simulink model "gm_hybrid_lht_vnl"  (R2019b)
settings: Solver=FixedStepDiscrete  StartTime=0.0  StopTime=inf  FixedStep=1/120e6  RelTol=1e-3
undefined symbols (not defined in the file or in its folder): bt, height, nTheta, width
libraries: hdlsllib x252, simulink x168, hdlmdlgenlib x11, dspsrcs4 x1
(part 11 of 12)

== system gm_hybrid_lht_vnl/Hybrid LHT/Hybrid LHT Kernel/Gradient Kernel System/Hough Kernel/Look Ahead Hough/Look Ahead Hough Symmetric/Register Bank_instance2 ==
  Data In : Inport  OutDataTypeStr=int8  PortDimensions=1  SampleTime=8.33333333333333e-09
  Write Enable : Inport  Port=2  OutDataTypeStr=boolean  PortDimensions=1  SampleTime=8.33333333333333e-09
  Delay_Switch : Switch  Criteria=u2 ~= 0  Threshold=double(0)  OutDataTypeStr=int8  SampleTime=8.33333333333333e-09
  Unit Delay Enabled Synchronous_lowered : Delay  DelayLength=double(1)  InitialCondition=0  SampleTime=8.33333333333333e-09
  Data Out : Outport
  wires:
  Unit Delay Enabled Synchronous_lowered/1 -> Data Out/1, Delay_Switch/3
  Data In/1 -> Delay_Switch/1
  Write Enable/1 -> Delay_Switch/2
  Delay_Switch/1 -> Unit Delay Enabled Synchronous_lowered/1

== system gm_hybrid_lht_vnl/Hybrid LHT/Hybrid LHT Kernel/Gradient Kernel System/Hough Kernel/Look Ahead Hough/Look Ahead Hough Symmetric/Register Bank_instance20 ==
  Data In : Inport  OutDataTypeStr=int8  PortDimensions=1  SampleTime=8.33333333333333e-09
  Write Enable : Inport  Port=2  OutDataTypeStr=boolean  PortDimensions=1  SampleTime=8.33333333333333e-09
  Delay_Switch : Switch  Criteria=u2 ~= 0  Threshold=double(0)  OutDataTypeStr=int8  SampleTime=8.33333333333333e-09
  Unit Delay Enabled Synchronous_lowered : Delay  DelayLength=double(1)  InitialCondition=0  SampleTime=8.33333333333333e-09
  Data Out : Outport
  wires:
  Unit Delay Enabled Synchronous_lowered/1 -> Data Out/1, Delay_Switch/3
  Data In/1 -> Delay_Switch/1
  Write Enable/1 -> Delay_Switch/2
  Delay_Switch/1 -> Unit Delay Enabled Synchronous_lowered/1

== system gm_hybrid_lht_vnl/Hybrid LHT/Hybrid LHT Kernel/Gradient Kernel System/Hough Kernel/Look Ahead Hough/Look Ahead Hough Symmetric/Register Bank_instance21 ==
  Data In : Inport  OutDataTypeStr=int8  PortDimensions=1  SampleTime=8.33333333333333e-09
  Write Enable : Inport  Port=2  OutDataTypeStr=boolean  PortDimensions=1  SampleTime=8.33333333333333e-09
  Delay_Switch : Switch  Criteria=u2 ~= 0  Threshold=double(0)  OutDataTypeStr=int8  SampleTime=8.33333333333333e-09
  Unit Delay Enabled Synchronous_lowered : Delay  DelayLength=double(1)  InitialCondition=0  SampleTime=8.33333333333333e-09
  Data Out : Outport
  wires:
  Unit Delay Enabled Synchronous_lowered/1 -> Data Out/1, Delay_Switch/3
  Data In/1 -> Delay_Switch/1
  Write Enable/1 -> Delay_Switch/2
  Delay_Switch/1 -> Unit Delay Enabled Synchronous_lowered/1

== system gm_hybrid_lht_vnl/Hybrid LHT/Hybrid LHT Kernel/Gradient Kernel System/Hough Kernel/Look Ahead Hough/Look Ahead Hough Symmetric/Register Bank_instance22 ==
  Data In : Inport  OutDataTypeStr=int8  PortDimensions=1  SampleTime=8.33333333333333e-09
  Write Enable : Inport  Port=2  OutDataTypeStr=boolean  PortDimensions=1  SampleTime=8.33333333333333e-09
  Delay_Switch : Switch  Criteria=u2 ~= 0  Threshold=double(0)  OutDataTypeStr=int8  SampleTime=8.33333333333333e-09
  Unit Delay Enabled Synchronous_lowered : Delay  DelayLength=double(1)  InitialCondition=0  SampleTime=8.33333333333333e-09
  Data Out : Outport
  wires:
  Unit Delay Enabled Synchronous_lowered/1 -> Data Out/1, Delay_Switch/3
  Data In/1 -> Delay_Switch/1
  Write Enable/1 -> Delay_Switch/2
  Delay_Switch/1 -> Unit Delay Enabled Synchronous_lowered/1

== system gm_hybrid_lht_vnl/Hybrid LHT/Hybrid LHT Kernel/Gradient Kernel System/Hough Kernel/Look Ahead Hough/Look Ahead Hough Symmetric/Register Bank_instance23 ==
  Data In : Inport  OutDataTypeStr=int8  PortDimensions=1  SampleTime=8.33333333333333e-09
  Write Enable : Inport  Port=2  OutDataTypeStr=boolean  PortDimensions=1  SampleTime=8.33333333333333e-09
  Delay_Switch : Switch  Criteria=u2 ~= 0  Threshold=double(0)  OutDataTypeStr=int8  SampleTime=8.33333333333333e-09
  Unit Delay Enabled Synchronous_lowered : Delay  DelayLength=double(1)  InitialCondition=0  SampleTime=8.33333333333333e-09
  Data Out : Outport
  wires:
  Unit Delay Enabled Synchronous_lowered/1 -> Data Out/1, Delay_Switch/3
  Data In/1 -> Delay_Switch/1
  Write Enable/1 -> Delay_Switch/2
  Delay_Switch/1 -> Unit Delay Enabled Synchronous_lowered/1

== system gm_hybrid_lht_vnl/Hybrid LHT/Hybrid LHT Kernel/Gradient Kernel System/Hough Kernel/Look Ahead Hough/Look Ahead Hough Symmetric/Register Bank_instance24 ==
  Data In : Inport  OutDataTypeStr=int8  PortDimensions=1  SampleTime=8.33333333333333e-09
  Write Enable : Inport  Port=2  OutDataTypeStr=boolean  PortDimensions=1  SampleTime=8.33333333333333e-09
  Delay_Switch : Switch  Criteria=u2 ~= 0  Threshold=double(0)  OutDataTypeStr=int8  SampleTime=8.33333333333333e-09
  Unit Delay Enabled Synchronous_lowered : Delay  DelayLength=double(1)  InitialCondition=0  SampleTime=8.33333333333333e-09
  Data Out : Outport
  wires:
  Unit Delay Enabled Synchronous_lowered/1 -> Data Out/1, Delay_Switch/3
  Data In/1 -> Delay_Switch/1
  Write Enable/1 -> Delay_Switch/2
  Delay_Switch/1 -> Unit Delay Enabled Synchronous_lowered/1

== system gm_hybrid_lht_vnl/Hybrid LHT/Hybrid LHT Kernel/Gradient Kernel System/Hough Kernel/Look Ahead Hough/Look Ahead Hough Symmetric/Register Bank_instance25 ==
  Data In : Inport  OutDataTypeStr=int8  PortDimensions=1  SampleTime=8.33333333333333e-09
  Write Enable : Inport  Port=2  OutDataTypeStr=boolean  PortDimensions=1  SampleTime=8.33333333333333e-09
  Delay_Switch : Switch  Criteria=u2 ~= 0  Threshold=double(0)  OutDataTypeStr=int8  SampleTime=8.33333333333333e-09
  Unit Delay Enabled Synchronous_lowered : Delay  DelayLength=double(1)  InitialCondition=0  SampleTime=8.33333333333333e-09
  Data Out : Outport
  wires:
  Unit Delay Enabled Synchronous_lowered/1 -> Data Out/1, Delay_Switch/3
  Data In/1 -> Delay_Switch/1
  Write Enable/1 -> Delay_Switch/2
  Delay_Switch/1 -> Unit Delay Enabled Synchronous_lowered/1

== system gm_hybrid_lht_vnl/Hybrid LHT/Hybrid LHT Kernel/Gradient Kernel System/Hough Kernel/Look Ahead Hough/Look Ahead Hough Symmetric/Register Bank_instance26 ==
  Data In : Inport  OutDataTypeStr=int8  PortDimensions=1  SampleTime=8.33333333333333e-09
  Write Enable : Inport  Port=2  OutDataTypeStr=boolean  PortDimensions=1  SampleTime=8.33333333333333e-09
  Delay_Switch : Switch  Criteria=u2 ~= 0  Threshold=double(0)  OutDataTypeStr=int8  SampleTime=8.33333333333333e-09
  Unit Delay Enabled Synchronous_lowered : Delay  DelayLength=double(1)  InitialCondition=0  SampleTime=8.33333333333333e-09
  Data Out : Outport
  wires:
  Unit Delay Enabled Synchronous_lowered/1 -> Data Out/1, Delay_Switch/3
  Data In/1 -> Delay_Switch/1
  Write Enable/1 -> Delay_Switch/2
  Delay_Switch/1 -> Unit Delay Enabled Synchronous_lowered/1

== system gm_hybrid_lht_vnl/Hybrid LHT/Hybrid LHT Kernel/Gradient Kernel System/Hough Kernel/Look Ahead Hough/Look Ahead Hough Symmetric/Register Bank_instance27 ==
  Data In : Inport  OutDataTypeStr=int8  PortDimensions=1  SampleTime=8.33333333333333e-09
  Write Enable : Inport  Port=2  OutDataTypeStr=boolean  PortDimensions=1  SampleTime=8.33333333333333e-09
  Delay_Switch : Switch  Criteria=u2 ~= 0  Threshold=double(0)  OutDataTypeStr=int8  SampleTime=8.33333333333333e-09
  Unit Delay Enabled Synchronous_lowered : Delay  DelayLength=double(1)  InitialCondition=0  SampleTime=8.33333333333333e-09
  Data Out : Outport
  wires:
  Unit Delay Enabled Synchronous_lowered/1 -> Data Out/1, Delay_Switch/3
  Data In/1 -> Delay_Switch/1
  Write Enable/1 -> Delay_Switch/2
  Delay_Switch/1 -> Unit Delay Enabled Synchronous_lowered/1

== system gm_hybrid_lht_vnl/Hybrid LHT/Hybrid LHT Kernel/Gradient Kernel System/Hough Kernel/Look Ahead Hough/Look Ahead Hough Symmetric/Register Bank_instance28 ==
  Data In : Inport  OutDataTypeStr=int8  PortDimensions=1  SampleTime=8.33333333333333e-09
  Write Enable : Inport  Port=2  OutDataTypeStr=boolean  PortDimensions=1  SampleTime=8.33333333333333e-09
  Delay_Switch : Switch  Criteria=u2 ~= 0  Threshold=double(0)  OutDataTypeStr=int8  SampleTime=8.33333333333333e-09
  Unit Delay Enabled Synchronous_lowered : Delay  DelayLength=double(1)  InitialCondition=0  SampleTime=8.33333333333333e-09
  Data Out : Outport
  wires:
  Unit Delay Enabled Synchronous_lowered/1 -> Data Out/1, Delay_Switch/3
  Data In/1 -> Delay_Switch/1
  Write Enable/1 -> Delay_Switch/2
  Delay_Switch/1 -> Unit Delay Enabled Synchronous_lowered/1

== system gm_hybrid_lht_vnl/Hybrid LHT/Hybrid LHT Kernel/Gradient Kernel System/Hough Kernel/Look Ahead Hough/Look Ahead Hough Symmetric/Register Bank_instance29 ==
  Data In : Inport  OutDataTypeStr=int8  PortDimensions=1  SampleTime=8.33333333333333e-09
  Write Enable : Inport  Port=2  OutDataTypeStr=boolean  PortDimensions=1  SampleTime=8.33333333333333e-09
  Delay_Switch : Switch  Criteria=u2 ~= 0  Threshold=double(0)  OutDataTypeStr=int8  SampleTime=8.33333333333333e-09
  Unit Delay Enabled Synchronous_lowered : Delay  DelayLength=double(1)  InitialCondition=0  SampleTime=8.33333333333333e-09
  Data Out : Outport
  wires:
  Unit Delay Enabled Synchronous_lowered/1 -> Data Out/1, Delay_Switch/3
  Data In/1 -> Delay_Switch/1
  Write Enable/1 -> Delay_Switch/2
  Delay_Switch/1 -> Unit Delay Enabled Synchronous_lowered/1

== system gm_hybrid_lht_vnl/Hybrid LHT/Hybrid LHT Kernel/Gradient Kernel System/Hough Kernel/Look Ahead Hough/Look Ahead Hough Symmetric/Register Bank_instance3 ==
  Data In : Inport  OutDataTypeStr=int8  PortDimensions=1  SampleTime=8.33333333333333e-09
  Write Enable : Inport  Port=2  OutDataTypeStr=boolean  PortDimensions=1  SampleTime=8.33333333333333e-09
  Delay_Switch : Switch  Criteria=u2 ~= 0  Threshold=double(0)  OutDataTypeStr=int8  SampleTime=8.33333333333333e-09
  Unit Delay Enabled Synchronous_lowered : Delay  DelayLength=double(1)  InitialCondition=0  SampleTime=8.33333333333333e-09
  Data Out : Outport
  wires:
  Delay_Switch/1 -> Unit Delay Enabled Synchronous_lowered/1
  Write Enable/1 -> Delay_Switch/2
  Data In/1 -> Delay_Switch/1
  Unit Delay Enabled Synchronous_lowered/1 -> Delay_Switch/3, Data Out/1

== system gm_hybrid_lht_vnl/Hybrid LHT/Hybrid LHT Kernel/Gradient Kernel System/Hough Kernel/Look Ahead Hough/Look Ahead Hough Symmetric/Register Bank_instance30 ==
  Data In : Inport  OutDataTypeStr=int8  PortDimensions=1  SampleTime=8.33333333333333e-09
  Write Enable : Inport  Port=2  OutDataTypeStr=boolean  PortDimensions=1  SampleTime=8.33333333333333e-09
  Delay_Switch : Switch  Criteria=u2 ~= 0  Threshold=double(0)  OutDataTypeStr=int8  SampleTime=8.33333333333333e-09
  Unit Delay Enabled Synchronous_lowered : Delay  DelayLength=double(1)  InitialCondition=0  SampleTime=8.33333333333333e-09
  Data Out : Outport
  wires:
  Unit Delay Enabled Synchronous_lowered/1 -> Data Out/1, Delay_Switch/3
  Data In/1 -> Delay_Switch/1
  Write Enable/1 -> Delay_Switch/2
  Delay_Switch/1 -> Unit Delay Enabled Synchronous_lowered/1

== system gm_hybrid_lht_vnl/Hybrid LHT/Hybrid LHT Kernel/Gradient Kernel System/Hough Kernel/Look Ahead Hough/Look Ahead Hough Symmetric/Register Bank_instance31 ==
  Data In : Inport  OutDataTypeStr=int8  PortDimensions=1  SampleTime=8.33333333333333e-09
  Write Enable : Inport  Port=2  OutDataTypeStr=boolean  PortDimensions=1  SampleTime=8.33333333333333e-09
  Delay_Switch : Switch  Criteria=u2 ~= 0  Threshold=double(0)  OutDataTypeStr=int8  SampleTime=8.33333333333333e-09
  Unit Delay Enabled Synchronous_lowered : Delay  DelayLength=double(1)  InitialCondition=0  SampleTime=8.33333333333333e-09
  Data Out : Outport
  wires:
  Unit Delay Enabled Synchronous_lowered/1 -> Data Out/1, Delay_Switch/3
  Data In/1 -> Delay_Switch/1
  Write Enable/1 -> Delay_Switch/2
  Delay_Switch/1 -> Unit Delay Enabled Synchronous_lowered/1

== system gm_hybrid_lht_vnl/Hybrid LHT/Hybrid LHT Kernel/Gradient Kernel System/Hough Kernel/Look Ahead Hough/Look Ahead Hough Symmetric/Register Bank_instance32 ==
  Data In : Inport  OutDataTypeStr=int8  PortDimensions=1  SampleTime=8.33333333333333e-09
  Write Enable : Inport  Port=2  OutDataTypeStr=boolean  PortDimensions=1  SampleTime=8.33333333333333e-09
  Delay_Switch : Switch  Criteria=u2 ~= 0  Threshold=double(0)  OutDataTypeStr=int8  SampleTime=8.33333333333333e-09
  Unit Delay Enabled Synchronous_lowered : Delay  DelayLength=double(1)  InitialCondition=0  SampleTime=8.33333333333333e-09
  Data Out : Outport
  wires:
  Unit Delay Enabled Synchronous_lowered/1 -> Data Out/1, Delay_Switch/3
  Data In/1 -> Delay_Switch/1
  Write Enable/1 -> Delay_Switch/2
  Delay_Switch/1 -> Unit Delay Enabled Synchronous_lowered/1

== system gm_hybrid_lht_vnl/Hybrid LHT/Hybrid LHT Kernel/Gradient Kernel System/Hough Kernel/Look Ahead Hough/Look Ahead Hough Symmetric/Register Bank_instance33 ==
  Data In : Inport  OutDataTypeStr=int8  PortDimensions=1  SampleTime=8.33333333333333e-09
  Write Enable : Inport  Port=2  OutDataTypeStr=boolean  PortDimensions=1  SampleTime=8.33333333333333e-09
  Delay_Switch : Switch  Criteria=u2 ~= 0  Threshold=double(0)  OutDataTypeStr=int8  SampleTime=8.33333333333333e-09
  Unit Delay Enabled Synchronous_lowered : Delay  DelayLength=double(1)  InitialCondition=0  SampleTime=8.33333333333333e-09
  Data Out : Outport
  wires:
  Unit Delay Enabled Synchronous_lowered/1 -> Data Out/1, Delay_Switch/3
  Data In/1 -> Delay_Switch/1
  Write Enable/1 -> Delay_Switch/2
  Delay_Switch/1 -> Unit Delay Enabled Synchronous_lowered/1

== system gm_hybrid_lht_vnl/Hybrid LHT/Hybrid LHT Kernel/Gradient Kernel System/Hough Kernel/Look Ahead Hough/Look Ahead Hough Symmetric/Register Bank_instance34 ==
  Data In : Inport  OutDataTypeStr=int8  PortDimensions=1  SampleTime=8.33333333333333e-09
  Write Enable : Inport  Port=2  OutDataTypeStr=boolean  PortDimensions=1  SampleTime=8.33333333333333e-09
  Delay_Switch : Switch  Criteria=u2 ~= 0  Threshold=double(0)  OutDataTypeStr=int8  SampleTime=8.33333333333333e-09
  Unit Delay Enabled Synchronous_lowered : Delay  DelayLength=double(1)  InitialCondition=0  SampleTime=8.33333333333333e-09
  Data Out : Outport
  wires:
  Unit Delay Enabled Synchronous_lowered/1 -> Data Out/1, Delay_Switch/3
  Data In/1 -> Delay_Switch/1
  Write Enable/1 -> Delay_Switch/2
  Delay_Switch/1 -> Unit Delay Enabled Synchronous_lowered/1

== system gm_hybrid_lht_vnl/Hybrid LHT/Hybrid LHT Kernel/Gradient Kernel System/Hough Kernel/Look Ahead Hough/Look Ahead Hough Symmetric/Register Bank_instance35 ==
  Data In : Inport  OutDataTypeStr=int8  PortDimensions=1  SampleTime=8.33333333333333e-09
  Write Enable : Inport  Port=2  OutDataTypeStr=boolean  PortDimensions=1  SampleTime=8.33333333333333e-09
  Delay_Switch : Switch  Criteria=u2 ~= 0  Threshold=double(0)  OutDataTypeStr=int8  SampleTime=8.33333333333333e-09
  Unit Delay Enabled Synchronous_lowered : Delay  DelayLength=double(1)  InitialCondition=0  SampleTime=8.33333333333333e-09
  Data Out : Outport
  wires:
  Unit Delay Enabled Synchronous_lowered/1 -> Data Out/1, Delay_Switch/3
  Data In/1 -> Delay_Switch/1
  Write Enable/1 -> Delay_Switch/2
  Delay_Switch/1 -> Unit Delay Enabled Synchronous_lowered/1

== system gm_hybrid_lht_vnl/Hybrid LHT/Hybrid LHT Kernel/Gradient Kernel System/Hough Kernel/Look Ahead Hough/Look Ahead Hough Symmetric/Register Bank_instance36 ==
  Data In : Inport  OutDataTypeStr=int8  PortDimensions=1  SampleTime=8.33333333333333e-09
  Write Enable : Inport  Port=2  OutDataTypeStr=boolean  PortDimensions=1  SampleTime=8.33333333333333e-09
  Delay_Switch : Switch  Criteria=u2 ~= 0  Threshold=double(0)  OutDataTypeStr=int8  SampleTime=8.33333333333333e-09
  Unit Delay Enabled Synchronous_lowered : Delay  DelayLength=double(1)  InitialCondition=0  SampleTime=8.33333333333333e-09
  Data Out : Outport
  wires:
  Unit Delay Enabled Synchronous_lowered/1 -> Data Out/1, Delay_Switch/3
  Data In/1 -> Delay_Switch/1
  Write Enable/1 -> Delay_Switch/2
  Delay_Switch/1 -> Unit Delay Enabled Synchronous_lowered/1

== system gm_hybrid_lht_vnl/Hybrid LHT/Hybrid LHT Kernel/Gradient Kernel System/Hough Kernel/Look Ahead Hough/Look Ahead Hough Symmetric/Register Bank_instance37 ==
  Data In : Inport  OutDataTypeStr=int8  PortDimensions=1  SampleTime=8.33333333333333e-09
  Write Enable : Inport  Port=2  OutDataTypeStr=boolean  PortDimensions=1  SampleTime=8.33333333333333e-09
  Delay_Switch : Switch  Criteria=u2 ~= 0  Threshold=double(0)  OutDataTypeStr=int8  SampleTime=8.33333333333333e-09
  Unit Delay Enabled Synchronous_lowered : Delay  DelayLength=double(1)  InitialCondition=0  SampleTime=8.33333333333333e-09
  Data Out : Outport
  wires:
  Unit Delay Enabled Synchronous_lowered/1 -> Data Out/1, Delay_Switch/3
  Data In/1 -> Delay_Switch/1
  Write Enable/1 -> Delay_Switch/2
  Delay_Switch/1 -> Unit Delay Enabled Synchronous_lowered/1

== system gm_hybrid_lht_vnl/Hybrid LHT/Hybrid LHT Kernel/Gradient Kernel System/Hough Kernel/Look Ahead Hough/Look Ahead Hough Symmetric/Register Bank_instance38 ==
  Data In : Inport  OutDataTypeStr=int8  PortDimensions=1  SampleTime=8.33333333333333e-09
  Write Enable : Inport  Port=2  OutDataTypeStr=boolean  PortDimensions=1  SampleTime=8.33333333333333e-09
  Delay_Switch : Switch  Criteria=u2 ~= 0  Threshold=double(0)  OutDataTypeStr=int8  SampleTime=8.33333333333333e-09
  Unit Delay Enabled Synchronous_lowered : Delay  DelayLength=double(1)  InitialCondition=0  SampleTime=8.33333333333333e-09
  Data Out : Outport
  wires:
  Unit Delay Enabled Synchronous_lowered/1 -> Data Out/1, Delay_Switch/3
  Data In/1 -> Delay_Switch/1
  Write Enable/1 -> Delay_Switch/2
  Delay_Switch/1 -> Unit Delay Enabled Synchronous_lowered/1

== system gm_hybrid_lht_vnl/Hybrid LHT/Hybrid LHT Kernel/Gradient Kernel System/Hough Kernel/Look Ahead Hough/Look Ahead Hough Symmetric/Register Bank_instance39 ==
  Data In : Inport  OutDataTypeStr=int8  PortDimensions=1  SampleTime=8.33333333333333e-09
  Write Enable : Inport  Port=2  OutDataTypeStr=boolean  PortDimensions=1  SampleTime=8.33333333333333e-09
  Delay_Switch : Switch  Criteria=u2 ~= 0  Threshold=double(0)  OutDataTypeStr=int8  SampleTime=8.33333333333333e-09
  Unit Delay Enabled Synchronous_lowered : Delay  DelayLength=double(1)  InitialCondition=0  SampleTime=8.33333333333333e-09
  Data Out : Outport
  wires:
  Unit Delay Enabled Synchronous_lowered/1 -> Data Out/1, Delay_Switch/3
  Data In/1 -> Delay_Switch/1
  Write Enable/1 -> Delay_Switch/2
  Delay_Switch/1 -> Unit Delay Enabled Synchronous_lowered/1

== system gm_hybrid_lht_vnl/Hybrid LHT/Hybrid LHT Kernel/Gradient Kernel System/Hough Kernel/Look Ahead Hough/Look Ahead Hough Symmetric/Register Bank_instance4 ==
  Data In : Inport  OutDataTypeStr=int8  PortDimensions=1  SampleTime=8.33333333333333e-09
  Write Enable : Inport  Port=2  OutDataTypeStr=boolean  PortDimensions=1  SampleTime=8.33333333333333e-09
  Delay_Switch : Switch  Criteria=u2 ~= 0  Threshold=double(0)  OutDataTypeStr=int8  SampleTime=8.33333333333333e-09
  Unit Delay Enabled Synchronous_lowered : Delay  DelayLength=double(1)  InitialCondition=0  SampleTime=8.33333333333333e-09
  Data Out : Outport
  wires:
  Unit Delay Enabled Synchronous_lowered/1 -> Data Out/1, Delay_Switch/3
  Data In/1 -> Delay_Switch/1
  Write Enable/1 -> Delay_Switch/2
  Delay_Switch/1 -> Unit Delay Enabled Synchronous_lowered/1

== system gm_hybrid_lht_vnl/Hybrid LHT/Hybrid LHT Kernel/Gradient Kernel System/Hough Kernel/Look Ahead Hough/Look Ahead Hough Symmetric/Register Bank_instance40 ==
  Data In : Inport  OutDataTypeStr=int8  PortDimensions=1  SampleTime=8.33333333333333e-09
  Write Enable : Inport  Port=2  OutDataTypeStr=boolean  PortDimensions=1  SampleTime=8.33333333333333e-09
  Delay_Switch : Switch  Criteria=u2 ~= 0  Threshold=double(0)  OutDataTypeStr=int8  SampleTime=8.33333333333333e-09
  Unit Delay Enabled Synchronous_lowered : Delay  DelayLength=double(1)  InitialCondition=0  SampleTime=8.33333333333333e-09
  Data Out : Outport
  wires:
  Unit Delay Enabled Synchronous_lowered/1 -> Data Out/1, Delay_Switch/3
  Data In/1 -> Delay_Switch/1
  Write Enable/1 -> Delay_Switch/2
  Delay_Switch/1 -> Unit Delay Enabled Synchronous_lowered/1

== system gm_hybrid_lht_vnl/Hybrid LHT/Hybrid LHT Kernel/Gradient Kernel System/Hough Kernel/Look Ahead Hough/Look Ahead Hough Symmetric/Register Bank_instance41 ==
  Data In : Inport  OutDataTypeStr=int8  PortDimensions=1  SampleTime=8.33333333333333e-09
  Write Enable : Inport  Port=2  OutDataTypeStr=boolean  PortDimensions=1  SampleTime=8.33333333333333e-09
  Delay_Switch : Switch  Criteria=u2 ~= 0  Threshold=double(0)  OutDataTypeStr=int8  SampleTime=8.33333333333333e-09
  Unit Delay Enabled Synchronous_lowered : Delay  DelayLength=double(1)  InitialCondition=0  SampleTime=8.33333333333333e-09
  Data Out : Outport
  wires:
  Unit Delay Enabled Synchronous_lowered/1 -> Data Out/1, Delay_Switch/3
  Data In/1 -> Delay_Switch/1
  Write Enable/1 -> Delay_Switch/2
  Delay_Switch/1 -> Unit Delay Enabled Synchronous_lowered/1

== system gm_hybrid_lht_vnl/Hybrid LHT/Hybrid LHT Kernel/Gradient Kernel System/Hough Kernel/Look Ahead Hough/Look Ahead Hough Symmetric/Register Bank_instance42 ==
  Data In : Inport  OutDataTypeStr=int8  PortDimensions=1  SampleTime=8.33333333333333e-09
  Write Enable : Inport  Port=2  OutDataTypeStr=boolean  PortDimensions=1  SampleTime=8.33333333333333e-09
  Delay_Switch : Switch  Criteria=u2 ~= 0  Threshold=double(0)  OutDataTypeStr=int8  SampleTime=8.33333333333333e-09
  Unit Delay Enabled Synchronous_lowered : Delay  DelayLength=double(1)  InitialCondition=0  SampleTime=8.33333333333333e-09
  Data Out : Outport
  wires:
  Unit Delay Enabled Synchronous_lowered/1 -> Data Out/1, Delay_Switch/3
  Data In/1 -> Delay_Switch/1
  Write Enable/1 -> Delay_Switch/2
  Delay_Switch/1 -> Unit Delay Enabled Synchronous_lowered/1

== system gm_hybrid_lht_vnl/Hybrid LHT/Hybrid LHT Kernel/Gradient Kernel System/Hough Kernel/Look Ahead Hough/Look Ahead Hough Symmetric/Register Bank_instance43 ==
  Data In : Inport  OutDataTypeStr=int8  PortDimensions=1  SampleTime=8.33333333333333e-09
  Write Enable : Inport  Port=2  OutDataTypeStr=boolean  PortDimensions=1  SampleTime=8.33333333333333e-09
  Delay_Switch : Switch  Criteria=u2 ~= 0  Threshold=double(0)  OutDataTypeStr=int8  SampleTime=8.33333333333333e-09
  Unit Delay Enabled Synchronous_lowered : Delay  DelayLength=double(1)  InitialCondition=0  SampleTime=8.33333333333333e-09
  Data Out : Outport
  wires:
  Unit Delay Enabled Synchronous_lowered/1 -> Data Out/1, Delay_Switch/3
  Data In/1 -> Delay_Switch/1
  Write Enable/1 -> Delay_Switch/2
  Delay_Switch/1 -> Unit Delay Enabled Synchronous_lowered/1

== system gm_hybrid_lht_vnl/Hybrid LHT/Hybrid LHT Kernel/Gradient Kernel System/Hough Kernel/Look Ahead Hough/Look Ahead Hough Symmetric/Register Bank_instance44 ==
  Data In : Inport  OutDataTypeStr=int8  PortDimensions=1  SampleTime=8.33333333333333e-09
  Write Enable : Inport  Port=2  OutDataTypeStr=boolean  PortDimensions=1  SampleTime=8.33333333333333e-09
  Delay_Switch : Switch  Criteria=u2 ~= 0  Threshold=double(0)  OutDataTypeStr=int8  SampleTime=8.33333333333333e-09
  Unit Delay Enabled Synchronous_lowered : Delay  DelayLength=double(1)  InitialCondition=0  SampleTime=8.33333333333333e-09
  Data Out : Outport
  wires:
  Unit Delay Enabled Synchronous_lowered/1 -> Data Out/1, Delay_Switch/3
  Data In/1 -> Delay_Switch/1
  Write Enable/1 -> Delay_Switch/2
  Delay_Switch/1 -> Unit Delay Enabled Synchronous_lowered/1

== system gm_hybrid_lht_vnl/Hybrid LHT/Hybrid LHT Kernel/Gradient Kernel System/Hough Kernel/Look Ahead Hough/Look Ahead Hough Symmetric/Register Bank_instance45 ==
  Data In : Inport  OutDataTypeStr=int8  PortDimensions=1  SampleTime=8.33333333333333e-09
  Write Enable : Inport  Port=2  OutDataTypeStr=boolean  PortDimensions=1  SampleTime=8.33333333333333e-09
  Delay_Switch : Switch  Criteria=u2 ~= 0  Threshold=double(0)  OutDataTypeStr=int8  SampleTime=8.33333333333333e-09
  Unit Delay Enabled Synchronous_lowered : Delay  DelayLength=double(1)  InitialCondition=0  SampleTime=8.33333333333333e-09
  Data Out : Outport
  wires:
  Unit Delay Enabled Synchronous_lowered/1 -> Data Out/1, Delay_Switch/3
  Data In/1 -> Delay_Switch/1
  Write Enable/1 -> Delay_Switch/2
  Delay_Switch/1 -> Unit Delay Enabled Synchronous_lowered/1

== system gm_hybrid_lht_vnl/Hybrid LHT/Hybrid LHT Kernel/Gradient Kernel System/Hough Kernel/Look Ahead Hough/Look Ahead Hough Symmetric/Register Bank_instance46 ==
  Data In : Inport  OutDataTypeStr=int8  PortDimensions=1  SampleTime=8.33333333333333e-09
  Write Enable : Inport  Port=2  OutDataTypeStr=boolean  PortDimensions=1  SampleTime=8.33333333333333e-09
  Delay_Switch : Switch  Criteria=u2 ~= 0  Threshold=double(0)  OutDataTypeStr=int8  SampleTime=8.33333333333333e-09
  Unit Delay Enabled Synchronous_lowered : Delay  DelayLength=double(1)  InitialCondition=0  SampleTime=8.33333333333333e-09
  Data Out : Outport
  wires:
  Unit Delay Enabled Synchronous_lowered/1 -> Data Out/1, Delay_Switch/3
  Data In/1 -> Delay_Switch/1
  Write Enable/1 -> Delay_Switch/2
  Delay_Switch/1 -> Unit Delay Enabled Synchronous_lowered/1

== system gm_hybrid_lht_vnl/Hybrid LHT/Hybrid LHT Kernel/Gradient Kernel System/Hough Kernel/Look Ahead Hough/Look Ahead Hough Symmetric/Register Bank_instance47 ==
  Data In : Inport  OutDataTypeStr=int8  PortDimensions=1  SampleTime=8.33333333333333e-09
  Write Enable : Inport  Port=2  OutDataTypeStr=boolean  PortDimensions=1  SampleTime=8.33333333333333e-09
  Delay_Switch : Switch  Criteria=u2 ~= 0  Threshold=double(0)  OutDataTypeStr=int8  SampleTime=8.33333333333333e-09
  Unit Delay Enabled Synchronous_lowered : Delay  DelayLength=double(1)  InitialCondition=0  SampleTime=8.33333333333333e-09
  Data Out : Outport
  wires:
  Unit Delay Enabled Synchronous_lowered/1 -> Data Out/1, Delay_Switch/3
  Data In/1 -> Delay_Switch/1
  Write Enable/1 -> Delay_Switch/2
  Delay_Switch/1 -> Unit Delay Enabled Synchronous_lowered/1

== system gm_hybrid_lht_vnl/Hybrid LHT/Hybrid LHT Kernel/Gradient Kernel System/Hough Kernel/Look Ahead Hough/Look Ahead Hough Symmetric/Register Bank_instance48 ==
  Data In : Inport  OutDataTypeStr=int8  PortDimensions=1  SampleTime=8.33333333333333e-09
  Write Enable : Inport  Port=2  OutDataTypeStr=boolean  PortDimensions=1  SampleTime=8.33333333333333e-09
  Delay_Switch : Switch  Criteria=u2 ~= 0  Threshold=double(0)  OutDataTypeStr=int8  SampleTime=8.33333333333333e-09
  Unit Delay Enabled Synchronous_lowered : Delay  DelayLength=double(1)  InitialCondition=0  SampleTime=8.33333333333333e-09
  Data Out : Outport
  wires:
  Unit Delay Enabled Synchronous_lowered/1 -> Data Out/1, Delay_Switch/3
  Data In/1 -> Delay_Switch/1
  Write Enable/1 -> Delay_Switch/2
  Delay_Switch/1 -> Unit Delay Enabled Synchronous_lowered/1

== system gm_hybrid_lht_vnl/Hybrid LHT/Hybrid LHT Kernel/Gradient Kernel System/Hough Kernel/Look Ahead Hough/Look Ahead Hough Symmetric/Register Bank_instance49 ==
  Data In : Inport  OutDataTypeStr=int8  PortDimensions=1  SampleTime=8.33333333333333e-09
  Write Enable : Inport  Port=2  OutDataTypeStr=boolean  PortDimensions=1  SampleTime=8.33333333333333e-09
  Delay_Switch : Switch  Criteria=u2 ~= 0  Threshold=double(0)  OutDataTypeStr=int8  SampleTime=8.33333333333333e-09
  Unit Delay Enabled Synchronous_lowered : Delay  DelayLength=double(1)  InitialCondition=0  SampleTime=8.33333333333333e-09
  Data Out : Outport
  wires:
  Unit Delay Enabled Synchronous_lowered/1 -> Data Out/1, Delay_Switch/3
  Data In/1 -> Delay_Switch/1
  Write Enable/1 -> Delay_Switch/2
  Delay_Switch/1 -> Unit Delay Enabled Synchronous_lowered/1

== system gm_hybrid_lht_vnl/Hybrid LHT/Hybrid LHT Kernel/Gradient Kernel System/Hough Kernel/Look Ahead Hough/Look Ahead Hough Symmetric/Register Bank_instance5 ==
  Data In : Inport  OutDataTypeStr=int8  PortDimensions=1  SampleTime=8.33333333333333e-09
  Write Enable : Inport  Port=2  OutDataTypeStr=boolean  PortDimensions=1  SampleTime=8.33333333333333e-09
  Delay_Switch : Switch  Criteria=u2 ~= 0  Threshold=double(0)  OutDataTypeStr=int8  SampleTime=8.33333333333333e-09
  Unit Delay Enabled Synchronous_lowered : Delay  DelayLength=double(1)  InitialCondition=0  SampleTime=8.33333333333333e-09
  Data Out : Outport
  wires:
  Unit Delay Enabled Synchronous_lowered/1 -> Data Out/1, Delay_Switch/3
  Data In/1 -> Delay_Switch/1
  Write Enable/1 -> Delay_Switch/2
  Delay_Switch/1 -> Unit Delay Enabled Synchronous_lowered/1

== system gm_hybrid_lht_vnl/Hybrid LHT/Hybrid LHT Kernel/Gradient Kernel System/Hough Kernel/Look Ahead Hough/Look Ahead Hough Symmetric/Register Bank_instance50 ==
  Data In : Inport  OutDataTypeStr=int8  PortDimensions=1  SampleTime=8.33333333333333e-09
  Write Enable : Inport  Port=2  OutDataTypeStr=boolean  PortDimensions=1  SampleTime=8.33333333333333e-09
  Delay_Switch : Switch  Criteria=u2 ~= 0  Threshold=double(0)  OutDataTypeStr=int8  SampleTime=8.33333333333333e-09
  Unit Delay Enabled Synchronous_lowered : Delay  DelayLength=double(1)  InitialCondition=0  SampleTime=8.33333333333333e-09
  Data Out : Outport
  wires:
  Unit Delay Enabled Synchronous_lowered/1 -> Data Out/1, Delay_Switch/3
  Data In/1 -> Delay_Switch/1
  Write Enable/1 -> Delay_Switch/2
  Delay_Switch/1 -> Unit Delay Enabled Synchronous_lowered/1

== system gm_hybrid_lht_vnl/Hybrid LHT/Hybrid LHT Kernel/Gradient Kernel System/Hough Kernel/Look Ahead Hough/Look Ahead Hough Symmetric/Register Bank_instance51 ==
  Data In : Inport  OutDataTypeStr=int8  PortDimensions=1  SampleTime=8.33333333333333e-09
  Write Enable : Inport  Port=2  OutDataTypeStr=boolean  PortDimensions=1  SampleTime=8.33333333333333e-09
  Delay_Switch : Switch  Criteria=u2 ~= 0  Threshold=double(0)  OutDataTypeStr=int8  SampleTime=8.33333333333333e-09
  Unit Delay Enabled Synchronous_lowered : Delay  DelayLength=double(1)  InitialCondition=0  SampleTime=8.33333333333333e-09
  Data Out : Outport
  wires:
  Unit Delay Enabled Synchronous_lowered/1 -> Data Out/1, Delay_Switch/3
  Data In/1 -> Delay_Switch/1
  Write Enable/1 -> Delay_Switch/2
  Delay_Switch/1 -> Unit Delay Enabled Synchronous_lowered/1

== system gm_hybrid_lht_vnl/Hybrid LHT/Hybrid LHT Kernel/Gradient Kernel System/Hough Kernel/Look Ahead Hough/Look Ahead Hough Symmetric/Register Bank_instance52 ==
  Data In : Inport  OutDataTypeStr=int8  PortDimensions=1  SampleTime=8.33333333333333e-09
  Write Enable : Inport  Port=2  OutDataTypeStr=boolean  PortDimensions=1  SampleTime=8.33333333333333e-09
  Delay_Switch : Switch  Criteria=u2 ~= 0  Threshold=double(0)  OutDataTypeStr=int8  SampleTime=8.33333333333333e-09
  Unit Delay Enabled Synchronous_lowered : Delay  DelayLength=double(1)  InitialCondition=0  SampleTime=8.33333333333333e-09
  Data Out : Outport
  wires:
  Unit Delay Enabled Synchronous_lowered/1 -> Data Out/1, Delay_Switch/3
  Data In/1 -> Delay_Switch/1
  Write Enable/1 -> Delay_Switch/2
  Delay_Switch/1 -> Unit Delay Enabled Synchronous_lowered/1

== system gm_hybrid_lht_vnl/Hybrid LHT/Hybrid LHT Kernel/Gradient Kernel System/Hough Kernel/Look Ahead Hough/Look Ahead Hough Symmetric/Register Bank_instance53 ==
  Data In : Inport  OutDataTypeStr=int8  PortDimensions=1  SampleTime=8.33333333333333e-09
  Write Enable : Inport  Port=2  OutDataTypeStr=boolean  PortDimensions=1  SampleTime=8.33333333333333e-09
  Delay_Switch : Switch  Criteria=u2 ~= 0  Threshold=double(0)  OutDataTypeStr=int8  SampleTime=8.33333333333333e-09
  Unit Delay Enabled Synchronous_lowered : Delay  DelayLength=double(1)  InitialCondition=0  SampleTime=8.33333333333333e-09
  Data Out : Outport
  wires:
  Unit Delay Enabled Synchronous_lowered/1 -> Data Out/1, Delay_Switch/3
  Data In/1 -> Delay_Switch/1
  Write Enable/1 -> Delay_Switch/2
  Delay_Switch/1 -> Unit Delay Enabled Synchronous_lowered/1

== system gm_hybrid_lht_vnl/Hybrid LHT/Hybrid LHT Kernel/Gradient Kernel System/Hough Kernel/Look Ahead Hough/Look Ahead Hough Symmetric/Register Bank_instance54 ==
  Data In : Inport  OutDataTypeStr=int8  PortDimensions=1  SampleTime=8.33333333333333e-09
  Write Enable : Inport  Port=2  OutDataTypeStr=boolean  PortDimensions=1  SampleTime=8.33333333333333e-09
  Delay_Switch : Switch  Criteria=u2 ~= 0  Threshold=double(0)  OutDataTypeStr=int8  SampleTime=8.33333333333333e-09
  Unit Delay Enabled Synchronous_lowered : Delay  DelayLength=double(1)  InitialCondition=0  SampleTime=8.33333333333333e-09
  Data Out : Outport
  wires:
  Unit Delay Enabled Synchronous_lowered/1 -> Data Out/1, Delay_Switch/3
  Data In/1 -> Delay_Switch/1
  Write Enable/1 -> Delay_Switch/2
  Delay_Switch/1 -> Unit Delay Enabled Synchronous_lowered/1

== system gm_hybrid_lht_vnl/Hybrid LHT/Hybrid LHT Kernel/Gradient Kernel System/Hough Kernel/Look Ahead Hough/Look Ahead Hough Symmetric/Register Bank_instance55 ==
  Data In : Inport  OutDataTypeStr=int8  PortDimensions=1  SampleTime=8.33333333333333e-09
  Write Enable : Inport  Port=2  OutDataTypeStr=boolean  PortDimensions=1  SampleTime=8.33333333333333e-09
  Delay_Switch : Switch  Criteria=u2 ~= 0  Threshold=double(0)  OutDataTypeStr=int8  SampleTime=8.33333333333333e-09
  Unit Delay Enabled Synchronous_lowered : Delay  DelayLength=double(1)  InitialCondition=0  SampleTime=8.33333333333333e-09
  Data Out : Outport
  wires:
  Unit Delay Enabled Synchronous_lowered/1 -> Data Out/1, Delay_Switch/3
  Data In/1 -> Delay_Switch/1
  Write Enable/1 -> Delay_Switch/2
  Delay_Switch/1 -> Unit Delay Enabled Synchronous_lowered/1

== system gm_hybrid_lht_vnl/Hybrid LHT/Hybrid LHT Kernel/Gradient Kernel System/Hough Kernel/Look Ahead Hough/Look Ahead Hough Symmetric/Register Bank_instance56 ==
  Data In : Inport  OutDataTypeStr=int8  PortDimensions=1  SampleTime=8.33333333333333e-09
  Write Enable : Inport  Port=2  OutDataTypeStr=boolean  PortDimensions=1  SampleTime=8.33333333333333e-09
  Delay_Switch : Switch  Criteria=u2 ~= 0  Threshold=double(0)  OutDataTypeStr=int8  SampleTime=8.33333333333333e-09
  Unit Delay Enabled Synchronous_lowered : Delay  DelayLength=double(1)  InitialCondition=0  SampleTime=8.33333333333333e-09
  Data Out : Outport
  wires:
  Unit Delay Enabled Synchronous_lowered/1 -> Data Out/1, Delay_Switch/3
  Data In/1 -> Delay_Switch/1
  Write Enable/1 -> Delay_Switch/2
  Delay_Switch/1 -> Unit Delay Enabled Synchronous_lowered/1

== system gm_hybrid_lht_vnl/Hybrid LHT/Hybrid LHT Kernel/Gradient Kernel System/Hough Kernel/Look Ahead Hough/Look Ahead Hough Symmetric/Register Bank_instance57 ==
  Data In : Inport  OutDataTypeStr=int8  PortDimensions=1  SampleTime=8.33333333333333e-09
  Write Enable : Inport  Port=2  OutDataTypeStr=boolean  PortDimensions=1  SampleTime=8.33333333333333e-09
  Delay_Switch : Switch  Criteria=u2 ~= 0  Threshold=double(0)  OutDataTypeStr=int8  SampleTime=8.33333333333333e-09
  Unit Delay Enabled Synchronous_lowered : Delay  DelayLength=double(1)  InitialCondition=0  SampleTime=8.33333333333333e-09
  Data Out : Outport
  wires:
  Unit Delay Enabled Synchronous_lowered/1 -> Data Out/1, Delay_Switch/3
  Data In/1 -> Delay_Switch/1
  Write Enable/1 -> Delay_Switch/2
  Delay_Switch/1 -> Unit Delay Enabled Synchronous_lowered/1

== system gm_hybrid_lht_vnl/Hybrid LHT/Hybrid LHT Kernel/Gradient Kernel System/Hough Kernel/Look Ahead Hough/Look Ahead Hough Symmetric/Register Bank_instance58 ==
  Data In : Inport  OutDataTypeStr=int8  PortDimensions=1  SampleTime=8.33333333333333e-09
  Write Enable : Inport  Port=2  OutDataTypeStr=boolean  PortDimensions=1  SampleTime=8.33333333333333e-09
  Delay_Switch : Switch  Criteria=u2 ~= 0  Threshold=double(0)  OutDataTypeStr=int8  SampleTime=8.33333333333333e-09
  Unit Delay Enabled Synchronous_lowered : Delay  DelayLength=double(1)  InitialCondition=0  SampleTime=8.33333333333333e-09
  Data Out : Outport
  wires:
  Unit Delay Enabled Synchronous_lowered/1 -> Data Out/1, Delay_Switch/3
  Data In/1 -> Delay_Switch/1
  Write Enable/1 -> Delay_Switch/2
  Delay_Switch/1 -> Unit Delay Enabled Synchronous_lowered/1

== system gm_hybrid_lht_vnl/Hybrid LHT/Hybrid LHT Kernel/Gradient Kernel System/Hough Kernel/Look Ahead Hough/Look Ahead Hough Symmetric/Register Bank_instance59 ==
  Data In : Inport  OutDataTypeStr=int8  PortDimensions=1  SampleTime=8.33333333333333e-09
  Write Enable : Inport  Port=2  OutDataTypeStr=boolean  PortDimensions=1  SampleTime=8.33333333333333e-09
  Delay_Switch : Switch  Criteria=u2 ~= 0  Threshold=double(0)  OutDataTypeStr=int8  SampleTime=8.33333333333333e-09
  Unit Delay Enabled Synchronous_lowered : Delay  DelayLength=double(1)  InitialCondition=0  SampleTime=8.33333333333333e-09
  Data Out : Outport
  wires:
  Unit Delay Enabled Synchronous_lowered/1 -> Data Out/1, Delay_Switch/3
  Data In/1 -> Delay_Switch/1
  Write Enable/1 -> Delay_Switch/2
  Delay_Switch/1 -> Unit Delay Enabled Synchronous_lowered/1

== system gm_hybrid_lht_vnl/Hybrid LHT/Hybrid LHT Kernel/Gradient Kernel System/Hough Kernel/Look Ahead Hough/Look Ahead Hough Symmetric/Register Bank_instance6 ==
  Data In : Inport  OutDataTypeStr=int8  PortDimensions=1  SampleTime=8.33333333333333e-09
  Write Enable : Inport  Port=2  OutDataTypeStr=boolean  PortDimensions=1  SampleTime=8.33333333333333e-09
  Delay_Switch : Switch  Criteria=u2 ~= 0  Threshold=double(0)  OutDataTypeStr=int8  SampleTime=8.33333333333333e-09
  Unit Delay Enabled Synchronous_lowered : Delay  DelayLength=double(1)  InitialCondition=0  SampleTime=8.33333333333333e-09
  Data Out : Outport
  wires:
  Unit Delay Enabled Synchronous_lowered/1 -> Data Out/1, Delay_Switch/3
  Data In/1 -> Delay_Switch/1
  Write Enable/1 -> Delay_Switch/2
  Delay_Switch/1 -> Unit Delay Enabled Synchronous_lowered/1

== system gm_hybrid_lht_vnl/Hybrid LHT/Hybrid LHT Kernel/Gradient Kernel System/Hough Kernel/Look Ahead Hough/Look Ahead Hough Symmetric/Register Bank_instance60 ==
  Data In : Inport  OutDataTypeStr=int8  PortDimensions=1  SampleTime=8.33333333333333e-09
  Write Enable : Inport  Port=2  OutDataTypeStr=boolean  PortDimensions=1  SampleTime=8.33333333333333e-09
  Delay_Switch : Switch  Criteria=u2 ~= 0  Threshold=double(0)  OutDataTypeStr=int8  SampleTime=8.33333333333333e-09
  Unit Delay Enabled Synchronous_lowered : Delay  DelayLength=double(1)  InitialCondition=0  SampleTime=8.33333333333333e-09
  Data Out : Outport
  wires:
  Unit Delay Enabled Synchronous_lowered/1 -> Data Out/1, Delay_Switch/3
  Data In/1 -> Delay_Switch/1
  Write Enable/1 -> Delay_Switch/2
  Delay_Switch/1 -> Unit Delay Enabled Synchronous_lowered/1

== system gm_hybrid_lht_vnl/Hybrid LHT/Hybrid LHT Kernel/Gradient Kernel System/Hough Kernel/Look Ahead Hough/Look Ahead Hough Symmetric/Register Bank_instance61 ==
  Data In : Inport  OutDataTypeStr=int8  PortDimensions=1  SampleTime=8.33333333333333e-09
  Write Enable : Inport  Port=2  OutDataTypeStr=boolean  PortDimensions=1  SampleTime=8.33333333333333e-09
  Delay_Switch : Switch  Criteria=u2 ~= 0  Threshold=double(0)  OutDataTypeStr=int8  SampleTime=8.33333333333333e-09
  Unit Delay Enabled Synchronous_lowered : Delay  DelayLength=double(1)  InitialCondition=0  SampleTime=8.33333333333333e-09
  Data Out : Outport
  wires:
  Unit Delay Enabled Synchronous_lowered/1 -> Data Out/1, Delay_Switch/3
  Data In/1 -> Delay_Switch/1
  Write Enable/1 -> Delay_Switch/2
  Delay_Switch/1 -> Unit Delay Enabled Synchronous_lowered/1

== system gm_hybrid_lht_vnl/Hybrid LHT/Hybrid LHT Kernel/Gradient Kernel System/Hough Kernel/Look Ahead Hough/Look Ahead Hough Symmetric/Register Bank_instance62 ==
  Data In : Inport  OutDataTypeStr=int8  PortDimensions=1  SampleTime=8.33333333333333e-09
  Write Enable : Inport  Port=2  OutDataTypeStr=boolean  PortDimensions=1  SampleTime=8.33333333333333e-09
  Delay_Switch : Switch  Criteria=u2 ~= 0  Threshold=double(0)  OutDataTypeStr=int8  SampleTime=8.33333333333333e-09
  Unit Delay Enabled Synchronous_lowered : Delay  DelayLength=double(1)  InitialCondition=0  SampleTime=8.33333333333333e-09
  Data Out : Outport
  wires:
  Unit Delay Enabled Synchronous_lowered/1 -> Data Out/1, Delay_Switch/3
  Data In/1 -> Delay_Switch/1
  Write Enable/1 -> Delay_Switch/2
  Delay_Switch/1 -> Unit Delay Enabled Synchronous_lowered/1

== system gm_hybrid_lht_vnl/Hybrid LHT/Hybrid LHT Kernel/Gradient Kernel System/Hough Kernel/Look Ahead Hough/Look Ahead Hough Symmetric/Register Bank_instance63 ==
  Data In : Inport  OutDataTypeStr=int8  PortDimensions=1  SampleTime=8.33333333333333e-09
  Write Enable : Inport  Port=2  OutDataTypeStr=boolean  PortDimensions=1  SampleTime=8.33333333333333e-09
  Delay_Switch : Switch  Criteria=u2 ~= 0  Threshold=double(0)  OutDataTypeStr=int8  SampleTime=8.33333333333333e-09
  Unit Delay Enabled Synchronous_lowered : Delay  DelayLength=double(1)  InitialCondition=0  SampleTime=8.33333333333333e-09
  Data Out : Outport
  wires:
  Unit Delay Enabled Synchronous_lowered/1 -> Data Out/1, Delay_Switch/3
  Data In/1 -> Delay_Switch/1
  Write Enable/1 -> Delay_Switch/2
  Delay_Switch/1 -> Unit Delay Enabled Synchronous_lowered/1

== system gm_hybrid_lht_vnl/Hybrid LHT/Hybrid LHT Kernel/Gradient Kernel System/Hough Kernel/Look Ahead Hough/Look Ahead Hough Symmetric/Register Bank_instance64 ==
  Data In : Inport  OutDataTypeStr=int8  PortDimensions=1  SampleTime=8.33333333333333e-09
  Write Enable : Inport  Port=2  OutDataTypeStr=boolean  PortDimensions=1  SampleTime=8.33333333333333e-09
  Delay_Switch : Switch  Criteria=u2 ~= 0  Threshold=double(0)  OutDataTypeStr=int8  SampleTime=8.33333333333333e-09
  Unit Delay Enabled Synchronous_lowered : Delay  DelayLength=double(1)  InitialCondition=0  SampleTime=8.33333333333333e-09
  Data Out : Outport
  wires:
  Unit Delay Enabled Synchronous_lowered/1 -> Data Out/1, Delay_Switch/3
  Data In/1 -> Delay_Switch/1
  Write Enable/1 -> Delay_Switch/2
  Delay_Switch/1 -> Unit Delay Enabled Synchronous_lowered/1

== system gm_hybrid_lht_vnl/Hybrid LHT/Hybrid LHT Kernel/Gradient Kernel System/Hough Kernel/Look Ahead Hough/Look Ahead Hough Symmetric/Register Bank_instance65 ==
  Data In : Inport  OutDataTypeStr=int8  PortDimensions=1  SampleTime=8.33333333333333e-09
  Write Enable : Inport  Port=2  OutDataTypeStr=boolean  PortDimensions=1  SampleTime=8.33333333333333e-09
  Delay_Switch : Switch  Criteria=u2 ~= 0  Threshold=double(0)  OutDataTypeStr=int8  SampleTime=8.33333333333333e-09
  Unit Delay Enabled Synchronous_lowered : Delay  DelayLength=double(1)  InitialCondition=0  SampleTime=8.33333333333333e-09
  Data Out : Outport
  wires:
  Unit Delay Enabled Synchronous_lowered/1 -> Data Out/1, Delay_Switch/3
  Data In/1 -> Delay_Switch/1
  Write Enable/1 -> Delay_Switch/2
  Delay_Switch/1 -> Unit Delay Enabled Synchronous_lowered/1

== system gm_hybrid_lht_vnl/Hybrid LHT/Hybrid LHT Kernel/Gradient Kernel System/Hough Kernel/Look Ahead Hough/Look Ahead Hough Symmetric/Register Bank_instance66 ==
  Data In : Inport  OutDataTypeStr=int8  PortDimensions=1  SampleTime=8.33333333333333e-09
  Write Enable : Inport  Port=2  OutDataTypeStr=boolean  PortDimensions=1  SampleTime=8.33333333333333e-09
  Delay_Switch : Switch  Criteria=u2 ~= 0  Threshold=double(0)  OutDataTypeStr=int8  SampleTime=8.33333333333333e-09
  Unit Delay Enabled Synchronous_lowered : Delay  DelayLength=double(1)  InitialCondition=0  SampleTime=8.33333333333333e-09
  Data Out : Outport
  wires:
  Unit Delay Enabled Synchronous_lowered/1 -> Data Out/1, Delay_Switch/3
  Data In/1 -> Delay_Switch/1
  Write Enable/1 -> Delay_Switch/2
  Delay_Switch/1 -> Unit Delay Enabled Synchronous_lowered/1

== system gm_hybrid_lht_vnl/Hybrid LHT/Hybrid LHT Kernel/Gradient Kernel System/Hough Kernel/Look Ahead Hough/Look Ahead Hough Symmetric/Register Bank_instance67 ==
  Data In : Inport  OutDataTypeStr=int8  PortDimensions=1  SampleTime=8.33333333333333e-09
  Write Enable : Inport  Port=2  OutDataTypeStr=boolean  PortDimensions=1  SampleTime=8.33333333333333e-09
  Delay_Switch : Switch  Criteria=u2 ~= 0  Threshold=double(0)  OutDataTypeStr=int8  SampleTime=8.33333333333333e-09
  Unit Delay Enabled Synchronous_lowered : Delay  DelayLength=double(1)  InitialCondition=0  SampleTime=8.33333333333333e-09
  Data Out : Outport
  wires:
  Unit Delay Enabled Synchronous_lowered/1 -> Data Out/1, Delay_Switch/3
  Data In/1 -> Delay_Switch/1
  Write Enable/1 -> Delay_Switch/2
  Delay_Switch/1 -> Unit Delay Enabled Synchronous_lowered/1

== system gm_hybrid_lht_vnl/Hybrid LHT/Hybrid LHT Kernel/Gradient Kernel System/Hough Kernel/Look Ahead Hough/Look Ahead Hough Symmetric/Register Bank_instance68 ==
  Data In : Inport  OutDataTypeStr=int8  PortDimensions=1  SampleTime=8.33333333333333e-09
  Write Enable : Inport  Port=2  OutDataTypeStr=boolean  PortDimensions=1  SampleTime=8.33333333333333e-09
  Delay_Switch : Switch  Criteria=u2 ~= 0  Threshold=double(0)  OutDataTypeStr=int8  SampleTime=8.33333333333333e-09
  Unit Delay Enabled Synchronous_lowered : Delay  DelayLength=double(1)  InitialCondition=0  SampleTime=8.33333333333333e-09
  Data Out : Outport
  wires:
  Unit Delay Enabled Synchronous_lowered/1 -> Data Out/1, Delay_Switch/3
  Data In/1 -> Delay_Switch/1
  Write Enable/1 -> Delay_Switch/2
  Delay_Switch/1 -> Unit Delay Enabled Synchronous_lowered/1

== system gm_hybrid_lht_vnl/Hybrid LHT/Hybrid LHT Kernel/Gradient Kernel System/Hough Kernel/Look Ahead Hough/Look Ahead Hough Symmetric/Register Bank_instance69 ==
  Data In : Inport  OutDataTypeStr=int8  PortDimensions=1  SampleTime=8.33333333333333e-09
  Write Enable : Inport  Port=2  OutDataTypeStr=boolean  PortDimensions=1  SampleTime=8.33333333333333e-09
  Delay_Switch : Switch  Criteria=u2 ~= 0  Threshold=double(0)  OutDataTypeStr=int8  SampleTime=8.33333333333333e-09
  Unit Delay Enabled Synchronous_lowered : Delay  DelayLength=double(1)  InitialCondition=0  SampleTime=8.33333333333333e-09
  Data Out : Outport
  wires:
  Unit Delay Enabled Synchronous_lowered/1 -> Data Out/1, Delay_Switch/3
  Data In/1 -> Delay_Switch/1
  Write Enable/1 -> Delay_Switch/2
  Delay_Switch/1 -> Unit Delay Enabled Synchronous_lowered/1

== system gm_hybrid_lht_vnl/Hybrid LHT/Hybrid LHT Kernel/Gradient Kernel System/Hough Kernel/Look Ahead Hough/Look Ahead Hough Symmetric/Register Bank_instance7 ==
  Data In : Inport  OutDataTypeStr=int8  PortDimensions=1  SampleTime=8.33333333333333e-09
  Write Enable : Inport  Port=2  OutDataTypeStr=boolean  PortDimensions=1  SampleTime=8.33333333333333e-09
  Delay_Switch : Switch  Criteria=u2 ~= 0  Threshold=double(0)  OutDataTypeStr=int8  SampleTime=8.33333333333333e-09
  Unit Delay Enabled Synchronous_lowered : Delay  DelayLength=double(1)  InitialCondition=0  SampleTime=8.33333333333333e-09
  Data Out : Outport
  wires:
  Unit Delay Enabled Synchronous_lowered/1 -> Data Out/1, Delay_Switch/3
  Data In/1 -> Delay_Switch/1
  Write Enable/1 -> Delay_Switch/2
  Delay_Switch/1 -> Unit Delay Enabled Synchronous_lowered/1

== system gm_hybrid_lht_vnl/Hybrid LHT/Hybrid LHT Kernel/Gradient Kernel System/Hough Kernel/Look Ahead Hough/Look Ahead Hough Symmetric/Register Bank_instance70 ==
  Data In : Inport  OutDataTypeStr=int8  PortDimensions=1  SampleTime=8.33333333333333e-09
  Write Enable : Inport  Port=2  OutDataTypeStr=boolean  PortDimensions=1  SampleTime=8.33333333333333e-09
  Delay_Switch : Switch  Criteria=u2 ~= 0  Threshold=double(0)  OutDataTypeStr=int8  SampleTime=8.33333333333333e-09
  Unit Delay Enabled Synchronous_lowered : Delay  DelayLength=double(1)  InitialCondition=0  SampleTime=8.33333333333333e-09
  Data Out : Outport
  wires:
  Unit Delay Enabled Synchronous_lowered/1 -> Data Out/1, Delay_Switch/3
  Data In/1 -> Delay_Switch/1
  Write Enable/1 -> Delay_Switch/2
  Delay_Switch/1 -> Unit Delay Enabled Synchronous_lowered/1

== system gm_hybrid_lht_vnl/Hybrid LHT/Hybrid LHT Kernel/Gradient Kernel System/Hough Kernel/Look Ahead Hough/Look Ahead Hough Symmetric/Register Bank_instance71 ==
  Data In : Inport  OutDataTypeStr=int8  PortDimensions=1  SampleTime=8.33333333333333e-09
  Write Enable : Inport  Port=2  OutDataTypeStr=boolean  PortDimensions=1  SampleTime=8.33333333333333e-09
  Delay_Switch : Switch  Criteria=u2 ~= 0  Threshold=double(0)  OutDataTypeStr=int8  SampleTime=8.33333333333333e-09
  Unit Delay Enabled Synchronous_lowered : Delay  DelayLength=double(1)  InitialCondition=0  SampleTime=8.33333333333333e-09
  Data Out : Outport
  wires:
  Unit Delay Enabled Synchronous_lowered/1 -> Data Out/1, Delay_Switch/3
  Data In/1 -> Delay_Switch/1
  Write Enable/1 -> Delay_Switch/2
  Delay_Switch/1 -> Unit Delay Enabled Synchronous_lowered/1

== system gm_hybrid_lht_vnl/Hybrid LHT/Hybrid LHT Kernel/Gradient Kernel System/Hough Kernel/Look Ahead Hough/Look Ahead Hough Symmetric/Register Bank_instance72 ==
  Data In : Inport  OutDataTypeStr=int8  PortDimensions=1  SampleTime=8.33333333333333e-09
  Write Enable : Inport  Port=2  OutDataTypeStr=boolean  PortDimensions=1  SampleTime=8.33333333333333e-09
  Delay_Switch : Switch  Criteria=u2 ~= 0  Threshold=double(0)  OutDataTypeStr=int8  SampleTime=8.33333333333333e-09
  Unit Delay Enabled Synchronous_lowered : Delay  DelayLength=double(1)  InitialCondition=0  SampleTime=8.33333333333333e-09
  Data Out : Outport
  wires:
  Unit Delay Enabled Synchronous_lowered/1 -> Data Out/1, Delay_Switch/3
  Data In/1 -> Delay_Switch/1
  Write Enable/1 -> Delay_Switch/2
  Delay_Switch/1 -> Unit Delay Enabled Synchronous_lowered/1
